simulink model "QPSK_HW_SW"  (R2017b)
settings: Solver=FixedStepDiscrete  StartTime=0.0  StopTime=inf  RelTol=1e-3
PreLoadFcn:
  | % Ensure SDR libraries are added to path
  | dev = sdrdev('PicoZed SDR');
  | dev.setupSession
  | clear dev; % clean up
  | 
  | sdrzQPSKTxFPGA_params = zynqRadioQPSKTxFPGAAD9361AD9364SL_init;
  | rcRolloff = 0.5;
  | sdrzQPSKrxFPGA = zynqRadioQPSKRxFPGAAD9361AD9364SL_init(rcRolloff);
  | % Need preamble & data from CST's QPSK Tx HDL example
  | qpsktxhdl=commqpsktxhdl_init();
  | 
  | % ARM Tx message
  | txtstr = '*Zynq HW/SW Codesign*';
InitFcn:
  | sdrzQPSKTxFPGA_params = zynqRadioQPSKTxFPGAAD9361AD9364SL_init;
  | rcRolloff = 0.5;
  | sdrzQPSKrxFPGA = zynqRadioQPSKRxFPGAAD9361AD9364SL_init(rcRolloff);
  | % Need preamble & data from CST's QPSK Tx HDL example
  | qpsktxhdl=commqpsktxhdl_init();
  | 
  | if (numel(txtstr) > 24)
  |   error('txtstr message must be less than 24 characters');
  | end;
undefined symbols (not defined in the file or in its folder): msglen
libraries: hdlsllib x15, dspsigops x6, commsequence2 x2, commdigbbndpm3 x2, dspmlti4 x2, commrandsrc3 x1, commutil2 x1, simulink x1, dspmathops x1
(part 1 of 2)
CloseFcn:
  | clear qpsktxhdl sdrzQPSKrxFPGA sdrzQPSKTxFPGA_params txtstr rcRolloff;
settings Model: DataTypeOverride=Off  Creator=The MathWorks, Inc.  LastModifiedBy=ppradhan
settings DataIOCC: SaveFormat=Array  SaveOutput=off  SaveTime=off
settings OptimizationCC: BlockReduction=off  ConditionallyExecuteInputs=off  DefaultParameterBehavior=Inlined  LifeSpan=inf
settings DebuggingCC: AlgebraicLoopMsg=error  SolverPrmCheckMsg=warning  SingleTaskRateTransMsg=error  ParameterPrecisionLossMsg=none  StrictBusMsg=ErrorOnBusTreatedAsVector  SFUnexpectedBacktrackingDiag=warning  SFNoUnconditionalDefaultTransitionDiag=warning  SFExecutionAtInitializationDiag=none
settings HardwareCC: ProdBitPerPointer=32  ProdBitPerSizeT=32  ProdBitPerPtrDiffT=32  ProdLargestAtomicFloat=None  ProdIntDivRoundTo=Undefined  ProdEndianess=Unspecified  ProdWordSize=32  ProdHWDeviceType=ASIC/FPGA->ASIC/FPGA  ProdEqTarget=off
settings ModelReferenceCC: PropagateSignalLabelsOutOfModel=off
settings CodeAppCC: StateflowObjectComments=on
settings GRTTargetCC: TargetLangStandard=C89/C90 (ANSI)  GeneratePreprocessorConditionals=Disable all
settings ConfigComp: CovMetricSettings=dw  CovHtmlReporting=on  CovSaveCumulativeToWorkspaceVar=on  CovSaveSingleToWorkspaceVar=on  CovExternalEMLEnable=off

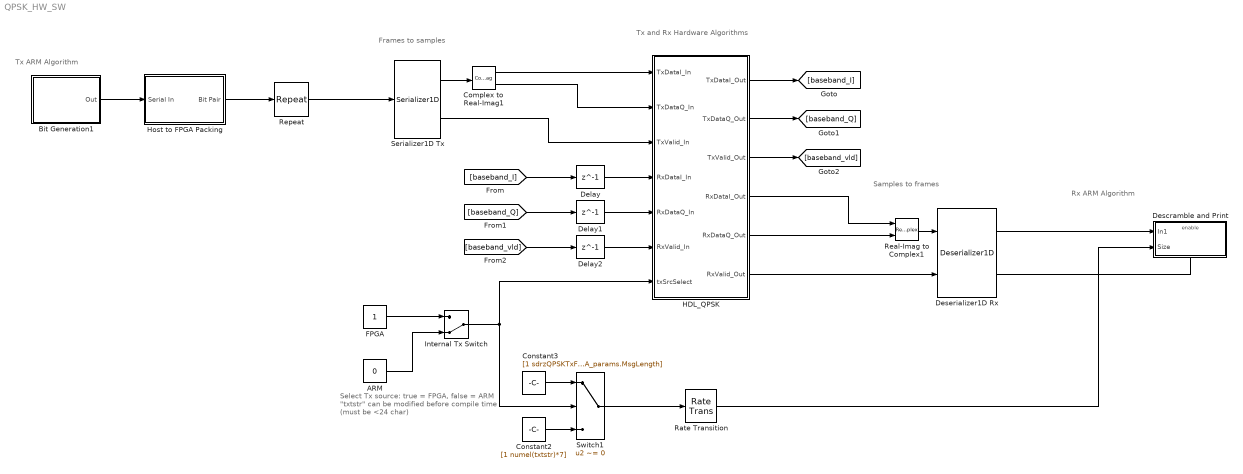
== system QPSK_HW_SW ==
  note: Select Tx source:
      | true = FPGA, false = ARM
      |
      | "txtstr" can be modified before
      | compile time (must be <24 char)
  note: Tx and Rx Hardware Algorithms
  note: Rx ARM Algorithm
  note: Samples to frames
  note: Frames to samples
  note: Tx ARM Algorithm
  ARM : Constant  Value=0  OutDataTypeStr=boolean  SampleTime=-1
  Bit Generation1 : Subsystem
      mask Display: disp('Bits Generation')
  Complex to Real-Imag1 : ComplexToRealImag
  Constant2 : Constant  Value=[1 numel(txtstr)*7]  SampleTime=-1
  Constant3 : Constant  Value=[1 sdrzQPSKTxFPGA_params.MsgLength]  SampleTime=-1
  Delay : Delay  DelayLength=1
  Delay1 : Delay  DelayLength=1
  Delay2 : Delay  DelayLength=1
  Descramble and Print : Subsystem  TreatAsAtomicUnit=on
  Deserializer1D Rx : hdlsllib/HDL Operations/Deserializer1D  Ratio=sdrzQPSKrxFPGA.FrameSize  IdleCycles=0  InitialCondition=0  startIn=off  validIn=on  validOut=on  inputDataDimensions=-1  inputSampleTime=-1  inputSignalType=auto
      settings: SourceProductName=HDL Coder  SourceProductBaseCode=HD
  FPGA : Constant  OutDataTypeStr=boolean  SampleTime=-1
  HDL_QPSK : Subsystem  TreatAsAtomicUnit=on
  Host to FPGA Packing : Subsystem
  Internal Tx Switch : ManualSwitch  CurrentSetting=0
  Rate Transition : RateTransition
  Real-Imag to Complex1 : RealImagToComplex
  Repeat : dspsigops/Repeat  N=4  InputProcessing=Columns as channels (frame based)  RateOptions=Allow multirate processing  ic=0  mode=Unused parameter value
      settings: SourceProductName=DSP System Toolbox
  Serializer1D Tx : hdlsllib/HDL Operations/Serializer1D  Ratio=200  IdleCycles=0  validIn=off  startOut=off  validOut=on  inputDataDimensions=-1  inputSampleTime=-1  inputSignalType=auto
      settings: SourceProductName=HDL Coder  SourceProductBaseCode=HD
  Switch1 : Switch  Criteria=u2 ~= 0
  wires:
  Deserializer1D Rx/1 -> Descramble and Print/1(In1)
  Real-Imag to Complex1/1 -> Deserializer1D Rx/1
  Deserializer1D Rx/2 -> Descramble and Print/Enable
  HDL_QPSK/4(RxDataI_Out) -> Real-Imag to Complex1/1
  HDL_QPSK/5(RxDataQ_Out) -> Real-Imag to Complex1/2
  HDL_QPSK/6(RxValid_Out) -> Deserializer1D Rx/2
  HDL_QPSK/1(TxDataI_Out) -> [baseband_I]
  HDL_QPSK/2(TxDataQ_Out) -> [baseband_Q]
  HDL_QPSK/3(TxValid_Out) -> [baseband_vld]
  [baseband_I] -> Delay/1
  [baseband_Q] -> Delay1/1
  [baseband_vld] -> Delay2/1
  Delay/1 -> HDL_QPSK/4(RxDataI_In)
  Delay1/1 -> HDL_QPSK/5(RxDataQ_In)
  Delay2/1 -> HDL_QPSK/6(RxValid_In)
  Host to FPGA Packing/1(Bit Pair) -> Repeat/1
  Bit Generation1/1(Out) -> Host to FPGA Packing/1(Serial In)
  Repeat/1 -> Serializer1D Tx/1
  Serializer1D Tx/1 -> Complex to Real-Imag1/1
  Complex to Real-Imag1/1 -> HDL_QPSK/1(TxDataI_In)
  Complex to Real-Imag1/2 -> HDL_QPSK/2(TxDataQ_In)
  Serializer1D Tx/2 -> HDL_QPSK/3(TxValid_In)
  ARM/1 -> Internal Tx Switch/2
  FPGA/1 -> Internal Tx Switch/1
  Switch1/1 -> Rate Transition/1
  Internal Tx Switch/1 -> HDL_QPSK/7(txSrcSelect), Switch1/2
  Constant2/1 -> Switch1/3
  Constant3/1 -> Switch1/1
  Rate Transition/1 -> Descramble and Print/2(Size)

== system QPSK_HW_SW/Bit Generation1 ==
  note: Each data frame contains 26 bits header (For Sync Purpose) and 174 bits data bits which
      | contain the txtStr message.Scrambler is there to improve data transition density and
      |  frequency offset estimation.
  Barker Code SS : Subsystem
      mask Display: disp('Unipolar\nBarker Code')
  Frame Conversion : FrameConversion  InheritSamplingMode=off  OutFrame=Sample-based
  Matrix Concatenate : Concatenate  Mode=Multidimensional array
  Message Source : Subsystem
      mask Display: disp('Message\nSource')
  Repeat : dspsigops/Repeat  N=2  InputProcessing=Columns as channels (frame based)  RateOptions=Enforce single-rate processing  ic=0  mode=Unused parameter value
      settings: SourceProductName=DSP System Toolbox
  Scrambler : commsequence2/Scrambler  M=2  poly=[1 1 1 0 1]  iniStaSource=Dialog Parameter  ini_sta=[0 0 0 0]  resetViaPort=off
      settings: SourceProductName=Communications System Toolbox  SourceProductBaseCode=CM
  Out : Outport
  wires:
  Message Source/1(Out) -> Scrambler/1
  Scrambler/1 -> Matrix Concatenate/2
  Repeat/1 -> Matrix Concatenate/1
  Barker Code SS/1(Out) -> Repeat/1
  Matrix Concatenate/1 -> Frame Conversion/1
  Frame Conversion/1 -> Out/1

== system QPSK_HW_SW/Descramble and Print ==
  In1 : Inport
  Size : Inport  Port=2
  Enable : EnablePort  PropagateVarSize=During execution
  BitsToDecimal1 : MATLAB Function  TreatAsAtomicUnit=on
  DataFramer : MATLAB Function  TreatAsAtomicUnit=on
  Descrambling : Subsystem
      mask Display: disp('Descrambling')
  wires:
  DataFramer/1(dataOut) -> Descrambling/1(In)
  In1/1 -> DataFramer/1(dataIn)
  Descrambling/1(Out) -> BitsToDecimal1/1(u)
  Size/1 -> Descrambling/2(Size)

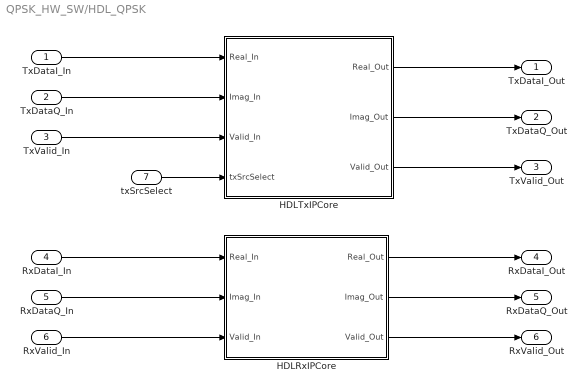
== system QPSK_HW_SW/HDL_QPSK ==
  TxDataI_In : Inport
  TxDataQ_In : Inport  Port=2
  TxValid_In : Inport  Port=3
  RxDataI_In : Inport  Port=4
  RxDataQ_In : Inport  Port=5
  RxValid_In : Inport  Port=6
  txSrcSelect : Inport  Port=7
  HDLRxIPCore : Subsystem  TreatAsAtomicUnit=on
  HDLTxIPCore : Subsystem  TreatAsAtomicUnit=on
  TxDataI_Out : Outport
  TxDataQ_Out : Outport  Port=2
  TxValid_Out : Outport  Port=3
  RxDataI_Out : Outport  Port=4
  RxDataQ_Out : Outport  Port=5
  RxValid_Out : Outport  Port=6
  wires:
  HDLTxIPCore/2(Imag_Out) -> TxDataQ_Out/1
  RxValid_In/1 -> HDLRxIPCore/3(Valid_In)
  HDLRxIPCore/3(Valid_Out) -> RxValid_Out/1
  HDLRxIPCore/2(Imag_Out) -> RxDataQ_Out/1
  HDLRxIPCore/1(Real_Out) -> RxDataI_Out/1
  HDLTxIPCore/3(Valid_Out) -> TxValid_Out/1
  RxDataQ_In/1 -> HDLRxIPCore/2(Imag_In)
  RxDataI_In/1 -> HDLRxIPCore/1(Real_In)
  HDLTxIPCore/1(Real_Out) -> TxDataI_Out/1
  TxDataI_In/1 -> HDLTxIPCore/1(Real_In)
  TxDataQ_In/1 -> HDLTxIPCore/2(Imag_In)
  TxValid_In/1 -> HDLTxIPCore/3(Valid_In)
  txSrcSelect/1 -> HDLTxIPCore/4(txSrcSelect)

== system QPSK_HW_SW/Host to FPGA Packing ==
  Serial In : Inport
  Data Type Conversion1 : DataTypeConversion  OutDataTypeStr=int16
  Downsample : DownSample  RateOptions=Allow multirate processing
  Downsample1 : DownSample  phase=1  RateOptions=Allow multirate processing
  Real-Imag to Complex : RealImagToComplex
  Bit Pair : Outport
  wires:
  Downsample/1 -> Real-Imag to Complex/1
  Serial In/1 -> Data Type Conversion1/1
  Data Type Conversion1/1 -> Downsample1/1, Downsample/1
  Downsample1/1 -> Real-Imag to Complex/2
  Real-Imag to Complex/1 -> Bit Pair/1

== system QPSK_HW_SW/Bit Generation1/Barker Code SS ==
  Constant Barker Code : Constant  Value=|  VectorParams1D=off  OutDataTypeStr=double
      | [+1 +1 +1 +1 +1 -1 -1 +1 +1 -1 +1 -1 +1
      | ].' > 0  % Bipolar to Unipolar Conversion
  Out : Outport
  wires:
  Constant Barker Code/1 -> Out/1

== system QPSK_HW_SW/Bit Generation1/Message Source ==
  Bernoulli Binary Generator : commrandsrc3/Bernoulli Binary Generator  ProbabilityOfZero=0.5  SeedSource=Parameter  Seed=61  SampleTime=sdrzQPSKTxFPGA_params.FrameTime / (sdrzQPSKTxFPGA_params.DataLength - numel(txtstr)*7)  SamplesPerFrame=sdrzQPSKTxFPGA_params.DataLength - numel(txtstr)*7  OutputDataType=double  SimulateUsing=Interpreted execution
  Integer to Bit Converter : commutil2/Integer to Bit Converter  nbits=7  signedInputValues=Unsigned  bitOrder=MSB first  outDtype=Inherit via internal rule
  Matrix Concatenate : Concatenate  Mode=Multidimensional array
  Scroll text : Constant  Value=double(txtstr)
  Out : Outport
  wires:
  Matrix Concatenate/1 -> Out/1
  Bernoulli Binary Generator/1 -> Matrix Concatenate/2
  Integer to Bit Converter/1 -> Matrix Concatenate/1
  Scroll text/1 -> Integer to Bit Converter/1

== system QPSK_HW_SW/Descramble and Print/Descrambling ==
  In : Inport
  Size : Inport  Port=2
  Descrambler : commsequence2/Descrambler  M=2  poly=[1 1 1 0 1]  iniStaSource=Dialog Parameter  ini_sta=[0 0 0 0]  resetViaPort=off
      settings: SourceProductName=Communications System Toolbox  SourceProductBaseCode=CM
  Selector : Selector  IndexOptions=Index vector (dialog)  Indices=[sdrzQPSKrxFPGA.BarkerLength*log2(sdrzQPSKrxFPGA.M)+1:sdrzQPSKrxFPGA.FrameSize*log2(sdrzQPSKrxFPGA.M)]  OutputSizes=1
  Selector1 : Selector  IndexOptions=Starting and ending indices (port)  Indices=[1:msglen]  OutputSizes=1
  Out : Outport
  wires:
  Selector/1 -> Descrambler/1
  In/1 -> Selector/1
  Selector1/1 -> Out/1
  Descrambler/1 -> Selector1/1
  Size/1 -> Selector1/2

== system QPSK_HW_SW/HDL_QPSK/HDLRxIPCore ==
  Real_In : Inport
  Imag_In : Inport  Port=2
  Valid_In : Inport  Port=3
  Complex to Real-Imag1 : ComplexToRealImag
  Enabled Delay : Delay  DelayLength=1  ShowEnablePort=on
      settings: InputPortMap=u0,e6
  HDLRx : Subsystem
  Real-Imag to Complex : RealImagToComplex
  Repeat : dspsigops/Repeat  N=sdrzQPSKrxFPGA.Upsampling/sdrzQPSKrxFPGA.Downsampling  InputProcessing=Columns as channels (frame based)  RateOptions=Allow multirate processing  ic=0  mode=Unused parameter value
      settings: SourceProductName=DSP System Toolbox
  Upsample : dspsigops/Upsample  N=sdrzQPSKrxFPGA.Upsampling/sdrzQPSKrxFPGA.Downsampling  phase=0  InputProcessing=Columns as channels (frame based)  RateOptions=Allow multirate processing  ic=0  mode=Unused parameter value
  Real_Out : Outport
  Imag_Out : Outport  Port=2
  Valid_Out : Outport  Port=3
  wires:
  HDLRx/2(dValidOut) -> Upsample/1
  Upsample/1 -> Valid_Out/1
  Repeat/1 -> Complex to Real-Imag1/1
  Complex to Real-Imag1/1 -> Real_Out/1
  Valid_In/1 -> Enabled Delay/2
  Complex to Real-Imag1/2 -> Imag_Out/1
  HDLRx/1(dataOutCh1) -> Repeat/1
  Real-Imag to Complex/1 -> Enabled Delay/1
  Enabled Delay/1 -> HDLRx/1(dataInCh1)
  Real_In/1 -> Real-Imag to Complex/1
  Imag_In/1 -> Real-Imag to Complex/2

== system QPSK_HW_SW/HDL_QPSK/HDLTxIPCore ==
  Real_In : Inport
  Imag_In : Inport  Port=2
  Valid_In : Inport  Port=3
  txSrcSelect : Inport  Port=4
  Complex to Real-Imag1 : ComplexToRealImag
  Delay : Delay  DelayLength=1
  Enabled Delay : Delay  DelayLength=1  ShowEnablePort=on
      settings: InputPortMap=u0,e6
  HDLTx : Subsystem
  Real-Imag to Complex : RealImagToComplex
  Real_Out : Outport
  Imag_Out : Outport  Port=2
  Valid_Out : Outport  Port=3
  wires:
  Complex to Real-Imag1/1 -> Real_Out/1
  Complex to Real-Imag1/2 -> Imag_Out/1
  HDLTx/1(dataoutCh1) -> Complex to Real-Imag1/1
  HDLTx/2(validoutCh1) -> Valid_Out/1
  Real-Imag to Complex/1 -> Enabled Delay/1
  Valid_In/1 -> HDLTx/2(validInCh1), Enabled Delay/2
  Real_In/1 -> Real-Imag to Complex/1
  Imag_In/1 -> Real-Imag to Complex/2
  Enabled Delay/1 -> HDLTx/1(dataInCh1)
  txSrcSelect/1 -> Delay/1
  Delay/1 -> HDLTx/3(txSrcSelect)

== system QPSK_HW_SW/HDL_QPSK/HDLRxIPCore/HDLRx ==
  dataInCh1 : Inport
  Automatic Gain Control : Subsystem  mask{AGCLoopGain=0.1, AGCUpperLimit=400, AGCRef=1/sqrt(sdrzQPSKrxFPGA.Upsampling)}
      mask prompts: AGCLoopGain "Loop Gain"; AGCUpperLimit "Maximum Gain"; AGCRef "Desired Amplitude"
  Coarse Frequency Compensation : Subsystem
  Data Decoding : Subsystem  TreatAsAtomicUnit=on  mask{Threshold=16}
      mask help:
      | Package synchronization is achieved by correlating (matched filtering) the Barker codes with the streams given by the Timing Recovery subsystem.
      | We deem successful package synchronization if the modulus of the matched filter output exceeds the threshold value defined below.
  FPGA to Host : Subsystem
  Fine Frequency Compensation : Subsystem
  Logical Operator1 : Logic  AllPortsSameDT=off  OutDataTypeStr=boolean
  Root Raised Cosine Receive Filter : dspmlti4/FIR Decimation  FilterSource=Dialog parameters  h=sdrzQPSKrxFPGA.rcRxFilt  D=sdrzQPSKrxFPGA.Upsampling/sdrzQPSKrxFPGA.Downsampling  filtStruct=Direct form  FilterObject=Hm_firdecim  framing=Allow multirate processing  inputOffset=0  outputBufInitCond=0  roundingMode=Floor  overflowMode=off  firstCoeffDataTypeStr=Inherit: Same word length as input  firstCoeffMin=[]  firstCoeffMax=[]  firstCoeffLastDataTypeStr=Inherit: Same word length as input  prodOutputMode=Binary point scaling  prodOutputWordLength=31  prodOutputFracLength=29  prodOutputDataTypeStr=fixdt(1,31,29)  prodOutputLastDataTypeStr=fixdt(1,31,29)  accumMode=Binary point scaling  accumWordLength=33  accumFracLength=29  accumDataTypeStr=fixdt(1,33,29)  accumLastDataTypeStr=fixdt(1,33,29)  outputMode=Binary point scaling  outputWordLength=16  outputFracLength=14  outputDataTypeStr=fixdt(1,16,14)  outputMin=[]  outputMax=[]  outputLastDataTypeStr=fixdt(1,16,14)
  Timing Recovery : Subsystem
  dataOutCh1 : Outport
  dValidOut : Outport  Port=2
  wires:
  FPGA to Host/1(Out) -> dataOutCh1/1
  Timing Recovery/2(DataOut) -> Data Decoding/1(In)
  dataInCh1/1 -> Automatic Gain Control/1(In)
  Fine Frequency Compensation/1(Out) -> Timing Recovery/1(In)
  Coarse Frequency Compensation/1(Out) -> Fine Frequency Compensation/1(In)
  Timing Recovery/1(dValid) -> Data Decoding/Enable, Logical Operator1/1
  Data Decoding/2(Bit1) -> FPGA to Host/1(bit1)
  Data Decoding/1(dValid) -> Logical Operator1/2
  Root Raised Cosine Receive Filter/1 -> Coarse Frequency Compensation/1(In)
  Automatic Gain Control/1(Out) -> Root Raised Cosine Receive Filter/1
  Logical Operator1/1 -> dValidOut/1
  Data Decoding/3(Bit2) -> FPGA to Host/2(bit2)

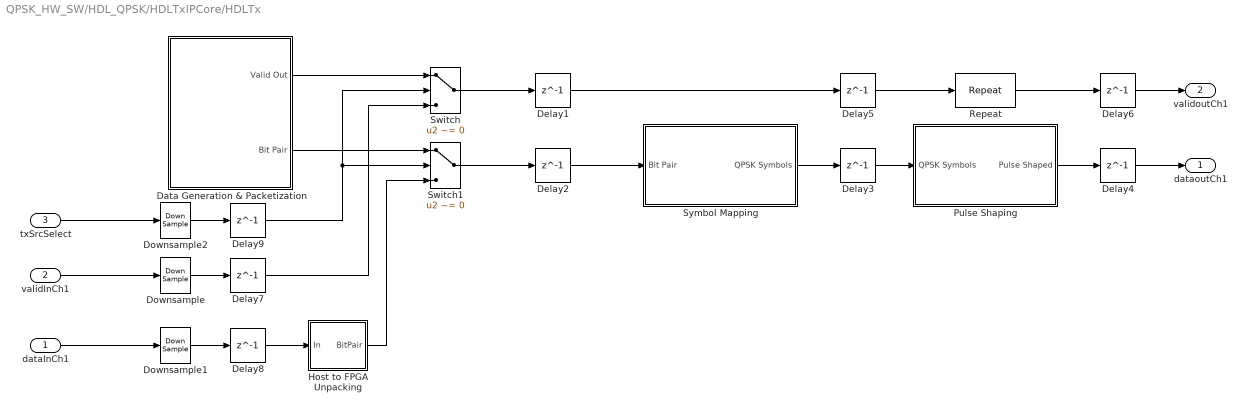
== system QPSK_HW_SW/HDL_QPSK/HDLTxIPCore/HDLTx ==
  dataInCh1 : Inport
  validInCh1 : Inport  Port=2
  txSrcSelect : Inport  Port=3
  Data Generation & Packetization : Subsystem
  Delay{1..9} (9 alike) : Delay  DelayLength=1  InitialCondition=0
  Downsample : DownSample  N=sdrzQPSKTxFPGA_params.Upsampling  RateOptions=Allow multirate processing
  Downsample1 : DownSample  N=sdrzQPSKTxFPGA_params.Upsampling  RateOptions=Allow multirate processing
  Downsample2 : DownSample  N=sdrzQPSKTxFPGA_params.Upsampling  RateOptions=Allow multirate processing
  Host to FPGA Unpacking : Subsystem
  Pulse Shaping : Subsystem
  Repeat : dspsigops/Repeat  N=sdrzQPSKTxFPGA_params.Upsampling  InputProcessing=Columns as channels (frame based)  RateOptions=Allow multirate processing  ic=0  mode=Unused parameter value
      settings: SourceProductName=DSP System Toolbox
  Switch : Switch  Criteria=u2 ~= 0
  Switch1 : Switch  Criteria=u2 ~= 0
  Symbol Mapping : Subsystem
  dataoutCh1 : Outport
  validoutCh1 : Outport  Port=2
  wires:
  Delay3/1 -> Pulse Shaping/1(QPSK Symbols)
  Pulse Shaping/1(Pulse Shaped) -> Delay4/1
  Delay4/1 -> dataoutCh1/1
  Delay2/1 -> Symbol Mapping/1(Bit Pair)
  Symbol Mapping/1(QPSK Symbols) -> Delay3/1
  Delay1/1 -> Delay5/1
  Delay5/1 -> Repeat/1
  Repeat/1 -> Delay6/1
  Delay6/1 -> validoutCh1/1
  Data Generation & Packetization/1(Valid Out) -> Switch/1
  Data Generation & Packetization/2(Bit Pair) -> Switch1/1
  Switch/1 -> Delay1/1
  Switch1/1 -> Delay2/1
  Downsample/1 -> Delay7/1
  Downsample1/1 -> Delay8/1
  validInCh1/1 -> Downsample/1
  dataInCh1/1 -> Downsample1/1
  Delay8/1 -> Host to FPGA Unpacking/1(In)
  Host to FPGA Unpacking/1(BitPair) -> Switch1/3
  Delay7/1 -> Switch/3
  Downsample2/1 -> Delay9/1
  txSrcSelect/1 -> Downsample2/1
  Delay9/1 -> Switch/2, Switch1/2

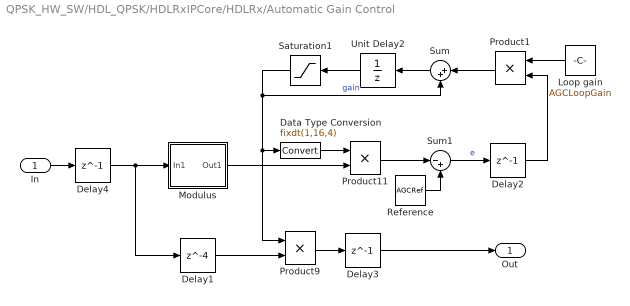
== system QPSK_HW_SW/HDL_QPSK/HDLRxIPCore/HDLRx/Automatic Gain Control ==
  In : Inport
  Data Type Conversion : DataTypeConversion  OutDataTypeStr=fixdt(1,16,4)  SaturateOnIntegerOverflow=on
  Delay1 : Delay  DelayLength=4  InitialCondition=0
  Delay2 : Delay  DelayLength=1  InitialCondition=0
  Delay3 : Delay  DelayLength=1  InitialCondition=0
  Delay4 : Delay  DelayLength=1  InitialCondition=0
  Loop gain : Constant  Value=AGCLoopGain  OutDataTypeStr=fixdt(1,16,10)  SampleTime=sdrzQPSKrxFPGA.Ts
  Modulus : Subsystem
  Product1 : Product  OutDataTypeStr=fixdt(1,16,10)  RndMeth=Zero
  Product11 : Product  OutDataTypeStr=fixdt(1,16,10)  RndMeth=Zero
  Product9 : Product  OutDataTypeStr=fixdt(1,16,14)  SaturateOnIntegerOverflow=on  RndMeth=Zero
  Reference : Constant  Value=AGCRef  OutDataTypeStr=fixdt(1,16,10)  SampleTime=sdrzQPSKrxFPGA.Ts
  Saturation1 : Saturate  UpperLimit=AGCUpperLimit  LowerLimit=1e-5
  Sum : Sum  Inputs=|++  OutDataTypeStr=fixdt(1,23,10)  SaturateOnIntegerOverflow=on
  Sum1 : Sum  Inputs=|-+  OutDataTypeStr=Inherit: Same as first input
  Unit Delay2 : UnitDelay  SampleTime=-1
  Out : Outport  PortDimensions=1
  wires:
  In/1 -> Delay4/1
  Product11/1 -> Sum1/1
  Data Type Conversion/1 -> Product11/1
  Reference/1 -> Sum1/2
  Sum/1 -> Unit Delay2/1
  Sum1/1 -> Delay2/1  "e"
  Product9/1 -> Delay3/1
  Delay1/1 -> Product9/2
  Delay3/1 -> Out/1
  Delay2/1 -> Product1/2
  Unit Delay2/1 -> Saturation1/1
  Delay4/1 -> Delay1/1, Modulus/1(In1)
  Modulus/1(Out1) -> Product11/2
  Product1/1 -> Sum/1
  Loop gain/1 -> Product1/1
  Saturation1/1 -> Data Type Conversion/1, Product9/1, Sum/2  "gain"

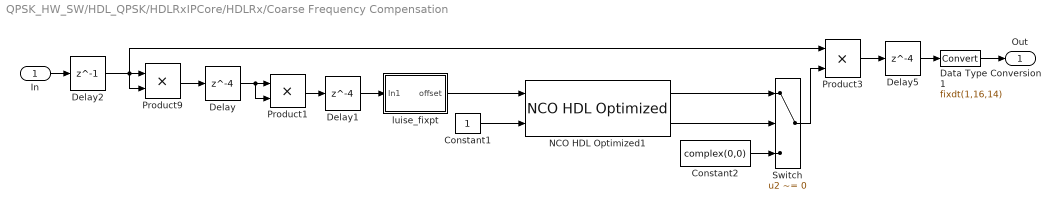
== system QPSK_HW_SW/HDL_QPSK/HDLRxIPCore/HDLRx/Coarse Frequency Compensation ==
  In : Inport  PortDimensions=1
  Constant1 : Constant  OutDataTypeStr=boolean  SampleTime=sdrzQPSKrxFPGA.Ts*sdrzQPSKrxFPGA.Upsampling/sdrzQPSKrxFPGA.Downsampling
  Constant2 : Constant  Value=complex(0,0)  OutDataTypeStr=fixdt(1,10,8)  SampleTime=sdrzQPSKrxFPGA.Ts*sdrzQPSKrxFPGA.Upsampling/sdrzQPSKrxFPGA.Downsampling
  Data Type Conversion1 : DataTypeConversion  OutDataTypeStr=fixdt(1,16,14)
  Delay : Delay  DelayLength=4  InitialCondition=0
  Delay1 : Delay  DelayLength=4  InitialCondition=0
  Delay2 : Delay  DelayLength=1  InitialCondition=0
  Delay5 : Delay  DelayLength=4  InitialCondition=0
  NCO HDL Optimized1 : dspsigops/NCO HDL Optimized  PhaseIncrementSource=Input port  PhaseIncrement=100  PhaseOffsetSource=Property  PhaseOffset=0  DitherSource=None  NumDitherBits=1  PhaseQuantization=on  NumQuantizerAccumulatorBits=16  LUTCompress=on  ResetAction=off  ValidInputPort=on  Waveform=Complex exponential  PhasePort=off  SimulateUsing=Code generation  AccumulatorWL=17  OutputDataType=Binary point scaling  OutputWL=10  OutputFL=8
      settings: SourceProductName=DSP System Toolbox  SourceProductBaseCode=DS
  Product1 : Product  SaturateOnIntegerOverflow=on  RndMeth=Zero
  Product3 : Product  SaturateOnIntegerOverflow=on  RndMeth=Zero
  Product9 : Product  OutDataTypeStr=fixdt(1,16,13)  SaturateOnIntegerOverflow=on  RndMeth=Zero
  Switch : Switch  Criteria=u2 ~= 0
  luise_fixpt : Subsystem
  Out : Outport
  wires:
  Data Type Conversion1/1 -> Out/1
  luise_fixpt/1(offset) -> NCO HDL Optimized1/1
  Delay1/1 -> luise_fixpt/1(In1)
  Product9/1 -> Delay/1
  Delay/1 -> Product1/1, Product1/2
  Product1/1 -> Delay1/1
  In/1 -> Delay2/1
  Product3/1 -> Delay5/1
  Delay5/1 -> Data Type Conversion1/1
  Constant1/1 -> NCO HDL Optimized1/2
  NCO HDL Optimized1/2 -> Switch/2
  NCO HDL Optimized1/1 -> Switch/1
  Constant2/1 -> Switch/3
  Switch/1 -> Product3/2
  Delay2/1 -> Product3/1, Product9/2, Product9/1

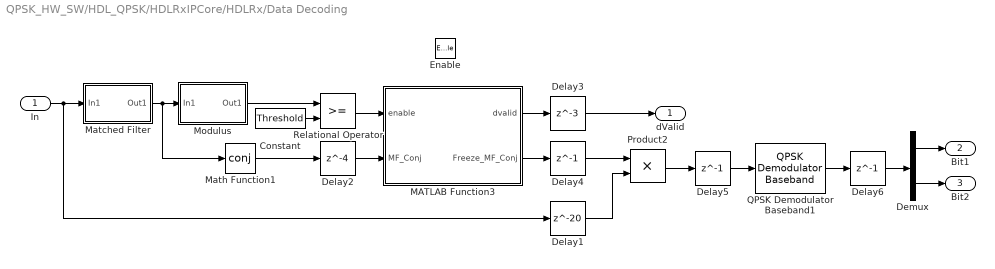
== system QPSK_HW_SW/HDL_QPSK/HDLRxIPCore/HDLRx/Data Decoding ==
  In : Inport
  Enable : EnablePort
  Constant : Constant  Value=Threshold  OutDataTypeStr=Inherit: Inherit via back propagation  SampleTime=sdrzQPSKrxFPGA.Ts*sdrzQPSKrxFPGA.Upsampling/sdrzQPSKrxFPGA.Downsampling
  Delay1 : Delay  DelayLength=20  InitialCondition=0
  Delay2 : Delay  DelayLength=4  InitialCondition=0
  Delay3 : Delay  DelayLength=3  InitialCondition=0
  Delay4 : Delay  DelayLength=1  InitialCondition=0
  Delay5 : Delay  DelayLength=1  InitialCondition=0
  Delay6 : Delay  DelayLength=1  InitialCondition=0
  Demux : Demux  Outputs=2
  MATLAB Function3 : MATLAB Function  TreatAsAtomicUnit=on
  Matched Filter : Subsystem
  Math Function1 : Math  Operator=conj  OutputSignalType=complex  SaturateOnIntegerOverflow=on
  Modulus : Subsystem
  Product2 : Product  SaturateOnIntegerOverflow=on  RndMeth=Zero
  QPSK Demodulator Baseband1 : commdigbbndpm3/QPSK Demodulator Baseband  OutType=Bit  DecType=Hard decision  VarSource=Dialog  Variance=1  Dec=Gray  Ph=pi/4  outDtype1=boolean  outDtype2=Inherit via internal rule  derotateFactorWordLen=16  derotateFactorDataTypeStr=Inherit: Same word length as input  derotateFactorLastDataTypeStr=Inherit: Same word length as input
  Relational Operator : RelationalOperator  OutDataTypeStr=boolean  RndMeth=Nearest  InputSameDT=on
  dValid : Outport  InitialOutput=0
  Bit1 : Outport  Port=2  InitialOutput=0
  Bit2 : Outport  Port=3  InitialOutput=0
  wires:
  Demux/2 -> Bit2/1
  Demux/1 -> Bit1/1
  Delay3/1 -> dValid/1
  Delay6/1 -> Demux/1
  Delay5/1 -> QPSK Demodulator Baseband1/1
  Delay1/1 -> Product2/2
  Delay4/1 -> Product2/1
  Delay2/1 -> MATLAB Function3/2(MF_Conj)
  Matched Filter/1(Out1) -> Math Function1/1, Modulus/1(In1)
  In/1 -> Delay1/1, Matched Filter/1(In1)
  Relational Operator/1 -> MATLAB Function3/1(enable)
  Math Function1/1 -> Delay2/1
  MATLAB Function3/2(Freeze_MF_Conj) -> Delay4/1
  MATLAB Function3/1(dvalid) -> Delay3/1
  QPSK Demodulator Baseband1/1 -> Delay6/1
  Modulus/1(Out1) -> Relational Operator/1
  Constant/1 -> Relational Operator/2
  Product2/1 -> Delay5/1

== system QPSK_HW_SW/HDL_QPSK/HDLRxIPCore/HDLRx/FPGA to Host ==
  bit1 : Inport
  bit2 : Inport  Port=2
  Data Type Conversion1 : DataTypeConversion  OutDataTypeStr=int16
  Data Type Conversion2 : DataTypeConversion  OutDataTypeStr=int16
  Real-Imag to Complex : RealImagToComplex
  Out : Outport
  wires:
  Data Type Conversion1/1 -> Real-Imag to Complex/1
  Real-Imag to Complex/1 -> Out/1
  bit2/1 -> Data Type Conversion2/1
  Data Type Conversion2/1 -> Real-Imag to Complex/2
  bit1/1 -> Data Type Conversion1/1

== system QPSK_HW_SW/HDL_QPSK/HDLRxIPCore/HDLRx/Fine Frequency Compensation ==
  In : Inport  PortDimensions=1
  Delay2 : Delay  InitialCondition=0
  Loop Filter : Subsystem  mask{BnTs=0.13, zeta=2.5, N=sdrzQPSKrxFPGA.Upsampling/sdrzQPSKrxFPGA.Downsampling}
      mask prompts: BnTs "Normalized Loop Bandwidth"; zeta "Damping Factor"; N "Number of Samples/Symbol"
      mask init:
      | % See C.57 to C.61 in Michael Rice's "Digital Communications 
      | % - A Discrete-Time Approach" for details
      | 
      | theta = BnTs/(zeta+0.25/zeta);  %0.0385
      | d = 1 + 2*zeta*theta + theta*theta; %1.1938
      | K1 = zeta*theta/d; %0.0805
      | K2 = theta*theta/(d*2); %6.1958e-04
      mask Display: disp('Loop Filter')
  MATLAB Function1 : MATLAB Function  TreatAsAtomicUnit=on
  Phase Calculation : Subsystem
  Product : Product  SaturateOnIntegerOverflow=on  OutDataTypeStr=Inherit: Same as first input
  Out : Outport
  wires:
  In/1 -> Product/1
  Loop Filter/1(v) -> Phase Calculation/1(Inc)
  MATLAB Function1/1(e) -> Loop Filter/1(e)
  Product/1 -> Delay2/1
  Delay2/1 -> MATLAB Function1/1(In), Out/1
  Phase Calculation/1(phShift) -> Product/2

== system QPSK_HW_SW/HDL_QPSK/HDLRxIPCore/HDLRx/Timing Recovery ==
  In : Inport
  Delay5 : Delay  DelayLength=6
  Integer Delay3 : Delay  DelayLength=1  InputProcessing=Inherited
  Integer Delay4 : Delay  DelayLength=1  InputProcessing=Inherited
  Interpolation Control : MATLAB Function
  Interpolation Filter : Subsystem
  Loop Filter : Subsystem  mask{BnTs=0.01, zeta=1, Kp=sdrzQPSKrxFPGA.TimingRecTEDGain, K0=sdrzQPSKrxFPGA.TimingRecCompensateGain, N=sdrzQPSKrxFPGA.Upsampling/sdrzQPSKrxFPGA.Downsampling}
      mask prompts: BnTs "Loop Bandwidth"; zeta "Loop Damping Factor"; Kp "Phase Detector Gain (Kp)"; K0 "DDS gain (K0)"; N "Number of Samples/symbol (N)"
      mask init:
      | % See C.57 to C.61 in Michael Rice's "Digital Communications 
      | % - A Discrete-Time Approach" for details
      | theta = BnTs/(zeta+0.25/zeta)/N;
      | d = 1 + 2*zeta*theta + theta*theta;
      | K1 = 4*zeta*theta/d;
      | K2 = 4*theta*theta/d;
      | K1 = K1/(Kp*K0);
      | K2 = K2/(Kp*K0);
      mask Display: disp('Loop Filter');
  Timing Error Detector : MATLAB Function  TreatAsAtomicUnit=on
  dValid : Outport
  DataOut : Outport  Port=2
  wires:
  Interpolation Filter/1(Out) -> Timing Error Detector/1(In), DataOut/1
  In/1 -> Delay5/1
  Integer Delay4/1 -> Interpolation Filter/2(mu)
  Interpolation Control/2(mu) -> Integer Delay4/1
  Interpolation Control/1(Underflow) -> Integer Delay3/1
  Delay5/1 -> Interpolation Filter/1(In)
  Integer Delay3/1 -> dValid/1, Timing Error Detector/2(strobe)
  Timing Error Detector/1(e) -> Loop Filter/1(e)
  Loop Filter/1(v) -> Interpolation Control/1(Delta)

== system QPSK_HW_SW/HDL_QPSK/HDLTxIPCore/HDLTx/Data Generation & Packetization ==
  Bit Pairing : Subsystem
  Data Source : Subsystem
  Downsample : DownSample  RateOptions=Allow multirate processing
  PacketizerFSM : MATLAB Function  TreatAsAtomicUnit=on  SystemSampleTime=1/sdrzQPSKrxFPGA.RadioFrontEndSampleRate*2
  Pipeline : Delay  InitialCondition=0
  Pipeline1 : Delay  DelayLength=1  InitialCondition=0
  Pipeline2 : Delay  DelayLength=1  InitialCondition=0
  Pipeline3 : Delay  DelayLength=1  InitialCondition=0
  Valid : Constant  OutDataTypeStr=boolean  SampleTime=1/sdrzQPSKrxFPGA.RadioFrontEndSampleRate*2
  Valid Out : Outport
  Bit Pair : Outport  Port=2
  wires:
  Bit Pairing/1(Bit Pair) -> Bit Pair/1
  Pipeline2/1 -> Bit Pairing/1(Serial In)
  Data Source/1(packets) -> Pipeline2/1
  Valid/1 -> Pipeline/1
  Pipeline1/1 -> Downsample/1
  Pipeline/1 -> Pipeline1/1
  Downsample/1 -> Pipeline3/1
  Pipeline3/1 -> Valid Out/1
  PacketizerFSM/1(reset_preamble) -> Data Source/1(reset preamble)
  PacketizerFSM/2(load_preamble) -> Data Source/2(load preamble)
  PacketizerFSM/3(load_data) -> Data Source/3(load data)

== system QPSK_HW_SW/HDL_QPSK/HDLTxIPCore/HDLTx/Host to FPGA Unpacking ==
  In : Inport
  Bit Concat : hdlsllib/HDL Operations/Bit Concat  numInputs=2
      settings: SourceProductName=HDL Coder  SourceProductBaseCode=HD
  Bit Slice1 : hdlsllib/HDL Operations/Bit Slice  lidx=0  ridx=0
      settings: SourceProductName=HDL Coder  SourceProductBaseCode=HD
  Bit Slice2 : hdlsllib/HDL Operations/Bit Slice  lidx=0  ridx=0
      settings: SourceProductName=HDL Coder  SourceProductBaseCode=HD
  Complex to Real-Imag : ComplexToRealImag
  BitPair : Outport
  wires:
  Complex to Real-Imag/1 -> Bit Slice2/1
  Complex to Real-Imag/2 -> Bit Slice1/1
  Bit Slice2/1 -> Bit Concat/1
  Bit Slice1/1 -> Bit Concat/2
  Bit Concat/1 -> BitPair/1
  In/1 -> Complex to Real-Imag/1

== system QPSK_HW_SW/HDL_QPSK/HDLTxIPCore/HDLTx/Pulse Shaping ==
  QPSK Symbols : Inport
  RRC Interpolation Filter : dspmlti4/FIR Interpolation  FilterSource=Dialog parameters  h=sdrzQPSKTxFPGA_params.TransmitterFilterCoefficients  L=sdrzQPSKTxFPGA_params.Upsampling  FilterObject=Htxrc  framing=Allow multirate processing  outputBufInitCond=0  roundingMode=Floor  overflowMode=off  firstCoeffMode=Specify word length  firstCoeffWordLength=16  firstCoeffFracLength=15  firstCoeffDataTypeStr=fixdt(1,16)  firstCoeffMin=[]  firstCoeffMax=[]  firstCoeffLastDataTypeStr=fixdt(1,16)  prodOutputMode=Binary point scaling  prodOutputWordLength=31  prodOutputFracLength=29  prodOutputDataTypeStr=fixdt(1,31,29)  prodOutputLastDataTypeStr=fixdt(1,31,29)  accumMode=Binary point scaling  accumWordLength=33  accumFracLength=29  accumDataTypeStr=fixdt(1,33,29)  accumLastDataTypeStr=fixdt(1,33,29)  outputMode=Binary point scaling  outputWordLength=16  outputFracLength=14  outputDataTypeStr=fixdt(1,16,14)  outputMin=[]  outputMax=[]  outputLastDataTypeStr=fixdt(1,16,14)
      settings: SourceProductName=DSP System Toolbox
  Pulse Shaped : Outport
  wires:
  QPSK Symbols/1 -> RRC Interpolation Filter/1
  RRC Interpolation Filter/1 -> Pulse Shaped/1

== system QPSK_HW_SW/HDL_QPSK/HDLTxIPCore/HDLTx/Symbol Mapping ==
  Bit Pair : Inport
  QPSK Modulator Baseband : commdigbbndpm3/QPSK Modulator Baseband  InType=Integer  Enc=Gray  Ph=pi/4  outDtype=Fixed-point  outWordLen=16  outUDDataType=sfix(16)  outFracLenMode=User-defined  outFracLen=15  outDataTypeStr=fixdt(1,16,15)  outLastDataTypeStr=fixdt(1,16,15)
  QPSK Symbols : Outport
  wires:
  QPSK Modulator Baseband/1 -> QPSK Symbols/1
  Bit Pair/1 -> QPSK Modulator Baseband/1

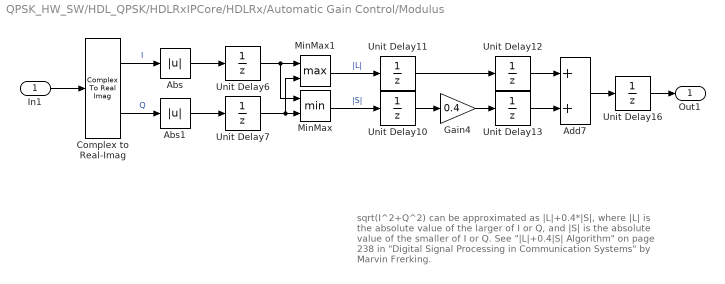
== system QPSK_HW_SW/HDL_QPSK/HDLRxIPCore/HDLRx/Automatic Gain Control/Modulus ==
  note: sqrt(I^2+Q^2) can be approximated as |L|+0.4*|S|,
      | where |L| is the absolute value of the larger of I or Q,
      | and |S| is the absolute value of the smaller of I or Q.
      |
      | See "|L|+0.4|S| Algorithm" on page 238 in "Digital Signal
      | Processing in Communication Systems" by Marvin Frerking.
  In1 : Inport
  Abs : Abs
  Abs1 : Abs
  Add7 : Sum
  Complex to Real-Imag : ComplexToRealImag
  Gain4 : Gain  Gain=0.4  OutDataTypeStr=fixdt(1,16,15)
  MinMax : MinMax  Inputs=2
  MinMax1 : MinMax  Function=max  Inputs=2
  Unit Delay{6..7,10..13,16} (7 alike) : UnitDelay  SampleTime=-1
  Out1 : Outport
  wires:
  Unit Delay11/1 -> Unit Delay12/1
  Unit Delay16/1 -> Out1/1
  Unit Delay10/1 -> Gain4/1
  Unit Delay12/1 -> Add7/1
  Abs1/1 -> Unit Delay7/1
  Add7/1 -> Unit Delay16/1
  Abs/1 -> Unit Delay6/1
  Complex to Real-Imag/1 -> Abs/1  "I"
  Complex to Real-Imag/2 -> Abs1/1  "Q"
  MinMax1/1 -> Unit Delay11/1  "|L|"
  Unit Delay13/1 -> Add7/2
  Gain4/1 -> Unit Delay13/1
  MinMax/1 -> Unit Delay10/1  "|S|"
  Unit Delay6/1 -> MinMax/1, MinMax1/1
  Unit Delay7/1 -> MinMax1/2, MinMax/2
  In1/1 -> Complex to Real-Imag/1

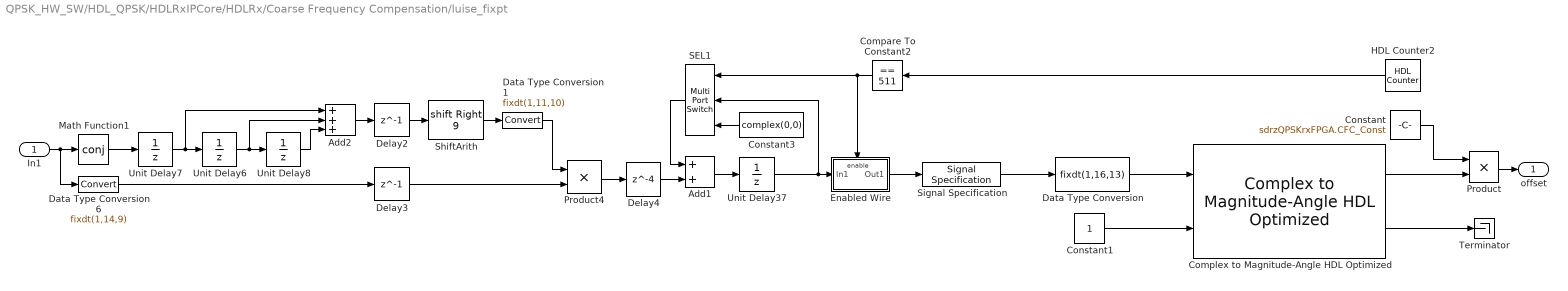
== system QPSK_HW_SW/HDL_QPSK/HDLRxIPCore/HDLRx/Coarse Frequency Compensation/luise_fixpt ==
  In1 : Inport
  Add1 : Sum  OutDataTypeStr=fixdt(1,33,20)
  Add2 : Sum  Inputs=+++  OutDataTypeStr=fixdt(1,33,20)
  Compare To Constant2 : simulink/Logic and Bit Operations/Compare To Constant  relop===  const=511  OutDataTypeStr=boolean
  Complex to Magnitude-Angle HDL Optimized : dspmathops/Complex to Magnitude-Angle HDL Optimized  NumIterationsSource=Property  NumIterations=5  OutputFormat=Angle  AngleFormat=Normalized  ScaleOutput=on  SimulateUsing=Code generation
      settings: SourceProductName=DSP System Toolbox  SourceProductBaseCode=DS
  Constant : Constant  Value=sdrzQPSKrxFPGA.CFC_Const  OutDataTypeStr=int16  SampleTime=sdrzQPSKrxFPGA.Ts*sdrzQPSKrxFPGA.Upsampling/sdrzQPSKrxFPGA.Downsampling
  Constant1 : Constant  OutDataTypeStr=boolean  SampleTime=sdrzQPSKrxFPGA.Ts*sdrzQPSKrxFPGA.Upsampling/sdrzQPSKrxFPGA.Downsampling
  Constant3 : Constant  Value=complex(0,0)  OutDataTypeStr=fixdt(1,16,14)  SampleTime=sdrzQPSKrxFPGA.Ts*sdrzQPSKrxFPGA.Upsampling/sdrzQPSKrxFPGA.Downsampling
  Data Type Conversion : DataTypeConversion  OutDataTypeStr=fixdt(1,16,13)
  Data Type Conversion1 : DataTypeConversion  OutDataTypeStr=fixdt(1,11,10)
  Data Type Conversion6 : DataTypeConversion  OutDataTypeStr=fixdt(1,14,9)  SaturateOnIntegerOverflow=on
  Delay2 : Delay  DelayLength=1  InitialCondition=0
  Delay3 : Delay  DelayLength=1  InitialCondition=0
  Delay4 : Delay  DelayLength=4  InitialCondition=0
  Enabled Wire : Subsystem  TreatAsAtomicUnit=on
  HDL Counter2 : hdlsllib/HDL Operations/HDL Counter  CountType=Count limited  CountInit=0  CountStep=1  CountMax=511  CountFromType=Initial value  CountFrom=0  CountResetPort=off  CountLoadPort=off  CountEnbPort=off  CountDirPort=off  CountDataType=Unsigned  CountWordLen=9  CountFracLen=0  CountSampTime=sdrzQPSKrxFPGA.Ts*sdrzQPSKrxFPGA.Upsampling/sdrzQPSKrxFPGA.Downsampling
      settings: SourceProductName=HDL Coder  SourceProductBaseCode=HD
  Math Function1 : Math  Operator=conj  OutputSignalType=complex  SaturateOnIntegerOverflow=on
  Product : Product  OutDataTypeStr=int16
  Product4 : Product  SaturateOnIntegerOverflow=on  RndMeth=Zero
  SEL1 : MultiPortSwitch  DataPortOrder=Zero-based contiguous  Inputs=2  DiagnosticForDefault=None  OutDataTypeStr=fixdt(1,33,20)
  ShiftArith : ArithShift  BitShiftNumber=9  BitShiftDirection=Right
  Signal Specification : SignalSpecification  Dimensions=1
  Terminator : Terminator
  Unit Delay37 : UnitDelay  InitialCondition=0+0j  SampleTime=-1
  Unit Delay6 : UnitDelay  SampleTime=-1
  Unit Delay7 : UnitDelay  SampleTime=-1
  Unit Delay8 : UnitDelay  SampleTime=-1
  offset : Outport  PortDimensions=1
  wires:
  Delay2/1 -> ShiftArith/1
  Delay3/1 -> Product4/2
  ShiftArith/1 -> Data Type Conversion1/1
  Unit Delay8/1 -> Add2/3
  HDL Counter2/1 -> Compare To Constant2/1
  Compare To Constant2/1 -> SEL1/1, Enabled Wire/Enable
  Unit Delay7/1 -> Unit Delay6/1, Add2/1
  Unit Delay6/1 -> Add2/2, Unit Delay8/1
  Constant3/1 -> SEL1/3
  Data Type Conversion6/1 -> Delay3/1
  Add2/1 -> Delay2/1
  SEL1/1 -> Add1/1
  Unit Delay37/1 -> SEL1/2, Enabled Wire/1(In1)
  Delay4/1 -> Add1/2
  Data Type Conversion1/1 -> Product4/1
  In1/1 -> Data Type Conversion6/1, Math Function1/1
  Product4/1 -> Delay4/1
  Math Function1/1 -> Unit Delay7/1
  Add1/1 -> Unit Delay37/1
  Enabled Wire/1(Out1) -> Signal Specification/1
  Product/1 -> offset/1
  Constant/1 -> Product/1
  Complex to Magnitude-Angle HDL Optimized/1 -> Product/2
  Constant1/1 -> Complex to Magnitude-Angle HDL Optimized/2
  Signal Specification/1 -> Data Type Conversion/1
  Complex to Magnitude-Angle HDL Optimized/2 -> Terminator/1
  Data Type Conversion/1 -> Complex to Magnitude-Angle HDL Optimized/1

== system QPSK_HW_SW/HDL_QPSK/HDLRxIPCore/HDLRx/Data Decoding/Matched Filter ==
  In1 : Inport
  Add2 : Sum
  Add3 : Sum  Inputs=+-
  Complex to Real-Imag2 : ComplexToRealImag
  Data Type Conversion1 : DataTypeConversion  OutDataTypeStr=fixdt(1,16,10)
  Data Type Conversion6 : DataTypeConversion  OutDataTypeStr=fixdt(1,16,10)
  Delay{1..4} (4 alike) : Delay  DelayLength=1  InitialCondition=0
  Discrete FIR Filter3 : DiscreteFir  FilterStructure=Direct form transposed  Coefficients=[-1 1 -1 1 -1 -1 1 1 -1 -1 -1 -1 -1]
  Discrete FIR Filter4 : DiscreteFir  FilterStructure=Direct form transposed  Coefficients=-1*[-1 1 -1 1 -1 -1 1 1 -1 -1 -1 -1 -1]
  Real-Imag to Complex2 : RealImagToComplex
  Out1 : Outport
  wires:
  Delay1/1 -> Discrete FIR Filter4/1
  Delay3/1 -> Real-Imag to Complex2/2
  Delay2/1 -> Real-Imag to Complex2/1
  Discrete FIR Filter4/1 -> Data Type Conversion1/1
  Delay4/1 -> Discrete FIR Filter3/1
  Discrete FIR Filter3/1 -> Data Type Conversion6/1
  Add3/1 -> Delay1/1
  Data Type Conversion6/1 -> Delay2/1
  Add2/1 -> Delay4/1
  Data Type Conversion1/1 -> Delay3/1
  Complex to Real-Imag2/1 -> Add3/1, Add2/1
  Complex to Real-Imag2/2 -> Add2/2, Add3/2
  Real-Imag to Complex2/1 -> Out1/1
  In1/1 -> Complex to Real-Imag2/1

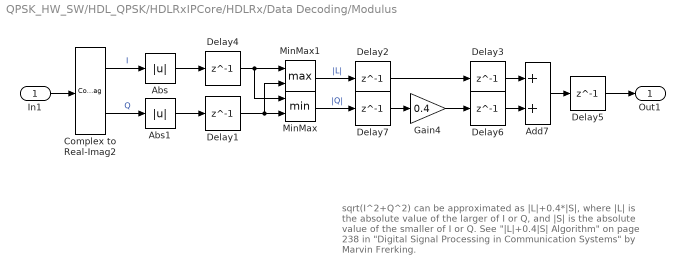
== system QPSK_HW_SW/HDL_QPSK/HDLRxIPCore/HDLRx/Data Decoding/Modulus ==
  note: sqrt(I^2+Q^2) can be approximated as |L|+0.4*|S|,
      | where |L| is the absolute value of the larger of I or Q,
      | and |S| is the absolute value of the smaller of I or Q.
      |
      | See "|L|+0.4|S| Algorithm" on page 238 in "Digital Signal
      | Processing in Communication Systems" by Marvin Frerking.
  In1 : Inport
  Abs : Abs
  Abs1 : Abs
  Add7 : Sum
  Complex to Real-Imag2 : ComplexToRealImag
  Delay{1..7} (7 alike) : Delay  DelayLength=1  InitialCondition=0
  Gain4 : Gain  Gain=0.4  OutDataTypeStr=fixdt(1,16,15)
  MinMax : MinMax  Inputs=2
  MinMax1 : MinMax  Function=max  Inputs=2
  Out1 : Outport
  wires:
  Complex to Real-Imag2/1 -> Abs/1  "I"
  Complex to Real-Imag2/2 -> Abs1/1  "Q"
  Delay3/1 -> Add7/1
  Delay5/1 -> Out1/1
  Delay6/1 -> Add7/2
  Delay4/1 -> MinMax/1, MinMax1/1
  Delay1/1 -> MinMax/2, MinMax1/2
  Delay2/1 -> Delay3/1
  Delay7/1 -> Gain4/1
  Add7/1 -> Delay5/1
  MinMax/1 -> Delay7/1  "|Q|"
  MinMax1/1 -> Delay2/1  "|L|"
  Gain4/1 -> Delay6/1
  Abs/1 -> Delay4/1
  Abs1/1 -> Delay1/1
  In1/1 -> Complex to Real-Imag2/1

== system QPSK_HW_SW/HDL_QPSK/HDLRxIPCore/HDLRx/Fine Frequency Compensation/Loop Filter ==
  note: Proportional-plus-Integrator Loop Filter,
      | Infinite DC Response to guarantee convergence
  e : Inport
  Data Type Conversion : DataTypeConversion  OutDataTypeStr=fixdt(1,16,15)
  Digital Filter : Subsystem
  K1 : Gain  Gain=K1  OutDataTypeStr=fixdt(1,16,15)
  K2 : Gain  Gain=K2  OutDataTypeStr=fixdt(1,32,32)
  Sum2 : Sum  OutDataTypeStr=fixdt(1,16,15)  SaturateOnIntegerOverflow=on
  Unit Delay2 : UnitDelay  SampleTime=-1
  v : Outport
  wires:
  Sum2/1 -> Unit Delay2/1
  Digital Filter/1(Out1) -> Data Type Conversion/1
  K1/1 -> Sum2/1
  Data Type Conversion/1 -> Sum2/2
  Unit Delay2/1 -> v/1
  e/1 -> K2/1, K1/1
  K2/1 -> Digital Filter/1(In1)

== system QPSK_HW_SW/HDL_QPSK/HDLRxIPCore/HDLRx/Fine Frequency Compensation/Phase Calculation ==
  Inc : Inport
  Add1 : Sum  OutDataTypeStr=fixdt(1,sdrzQPSKrxFPGA.WL_acc ,0)
  Constant : Constant  Value=sdrzQPSKrxFPGA.FFC_Const  OutDataTypeStr=fixdt(1,sdrzQPSKrxFPGA.WL_acc,0)  SampleTime=sdrzQPSKrxFPGA.Ts*sdrzQPSKrxFPGA.Upsampling/sdrzQPSKrxFPGA.Downsampling
  Integer Delay4 : Delay  DelayLength=1  InitialCondition=0  InputProcessing=Inherited
  Product : Product  OutDataTypeStr=fixdt(1,sdrzQPSKrxFPGA.WL_acc,0)
  Quart_Sin_Cos_LUT : Subsystem
  Real-Imag to Complex2 : RealImagToComplex
  Signal Specification : SignalSpecification  Dimensions=1
  phShift : Outport
  wires:
  Product/1 -> Add1/2
  Constant/1 -> Product/2
  Inc/1 -> Product/1
  Add1/1 -> Integer Delay4/1
  Integer Delay4/1 -> Add1/1, Signal Specification/1
  Quart_Sin_Cos_LUT/2(cosValue) -> Real-Imag to Complex2/1
  Quart_Sin_Cos_LUT/1(sineValue) -> Real-Imag to Complex2/2
  Real-Imag to Complex2/1 -> phShift/1
  Signal Specification/1 -> Quart_Sin_Cos_LUT/1(Phase)

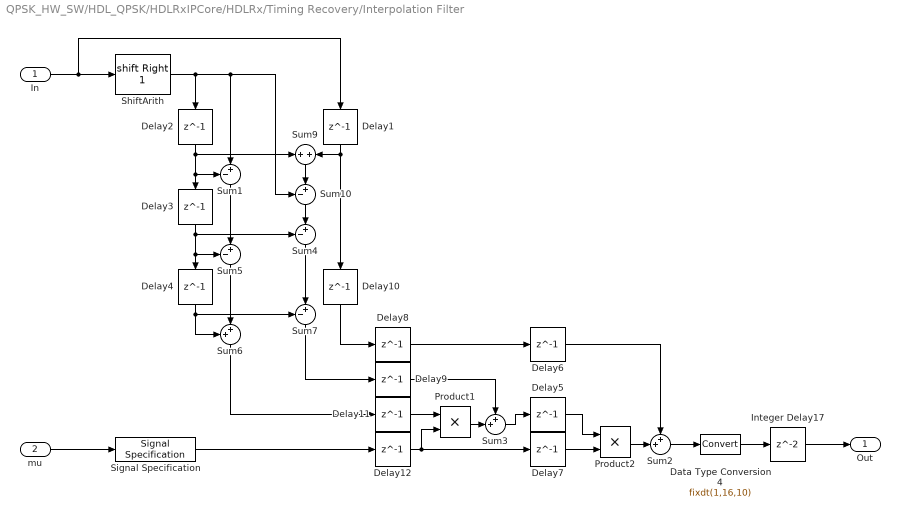
== system QPSK_HW_SW/HDL_QPSK/HDLRxIPCore/HDLRx/Timing Recovery/Interpolation Filter ==
  In : Inport
  mu : Inport  Port=2
  Data Type Conversion4 : DataTypeConversion  OutDataTypeStr=fixdt(1,16,10)
  Delay{1..12} (12 alike) : Delay  DelayLength=1  InitialCondition=0
  Integer Delay17 : Delay  InitialCondition=0  InputProcessing=Inherited
  Product1 : Product  OutDataTypeStr=fixdt(1,16,10)  RndMeth=Zero
  Product2 : Product  RndMeth=Zero
  ShiftArith : ArithShift  BitShiftNumber=1  BitShiftDirection=Right
  Signal Specification : SignalSpecification  Dimensions=1
  Sum{1,4..5,10} (4 alike) : Sum  Inputs=-+|
  Sum2 : Sum  Inputs=++|
  Sum3 : Sum  Inputs=++|  OutDataTypeStr=fixdt(1,16,10)
  Sum6 : Sum  Inputs=++|  OutDataTypeStr=fixdt(1,16,11)  SaturateOnIntegerOverflow=on
  Sum7 : Sum  Inputs=-+|  OutDataTypeStr=fixdt(1,16,10)
  Sum9 : Sum  Inputs=+|+
  Out : Outport
  wires:
  ShiftArith/1 -> Delay2/1, Sum1/2, Sum10/1
  Delay1/1 -> Sum9/2, Delay10/1
  Delay2/1 -> Sum9/1, Delay3/1, Sum1/1
  Sum10/1 -> Sum4/2
  Delay3/1 -> Delay4/1, Sum5/1, Sum4/1
  Sum1/1 -> Sum5/2
  Delay4/1 -> Sum6/1, Sum7/1
  Sum5/1 -> Sum6/2
  Sum4/1 -> Sum7/2
  Delay5/1 -> Product2/1
  Sum3/1 -> Delay5/1
  Product2/1 -> Sum2/2
  Product1/1 -> Sum3/2
  Sum2/1 -> Data Type Conversion4/1
  Delay11/1 -> Product1/1
  Delay9/1 -> Sum3/1
  Delay8/1 -> Delay6/1
  Delay12/1 -> Delay7/1, Product1/2
  Delay7/1 -> Product2/2
  Delay6/1 -> Sum2/1
  Delay10/1 -> Delay8/1
  Sum7/1 -> Delay9/1
  Sum6/1 -> Delay11/1
  mu/1 -> Signal Specification/1
  Integer Delay17/1 -> Out/1
  In/1 -> Delay1/1, ShiftArith/1
  Data Type Conversion4/1 -> Integer Delay17/1
  Sum9/1 -> Sum10/2
  Signal Specification/1 -> Delay12/1

== system QPSK_HW_SW/HDL_QPSK/HDLRxIPCore/HDLRx/Timing Recovery/Loop Filter ==
  note: Proportional-Plus-Integrator Loop Filter,
      | Infinite DC Response to guarantee convergence
  e : Inport
  Data Type Conversion17 : DataTypeConversion  OutDataTypeStr=fixdt(1,11,10)
  Delay1 : Delay  DelayLength=1  InitialCondition=0
  Delay2 : Delay  DelayLength=1  InitialCondition=0
  Delay4 : Delay  DelayLength=1  InitialCondition=0
  Digital Filter : Subsystem
  K1 : Gain  Gain=K1  OutDataTypeStr=fixdt(1,40,33)
  K2 : Gain  Gain=K2
  Sum2 : Sum  SaturateOnIntegerOverflow=on  InputSameDT=on
  v : Outport
  wires:
  e/1 -> Delay2/1
  Sum2/1 -> Data Type Conversion17/1
  Delay1/1 -> Sum2/1
  Delay4/1 -> Sum2/2
  Delay2/1 -> K1/1, K2/1
  Data Type Conversion17/1 -> v/1
  K2/1 -> Digital Filter/1(In1)
  Digital Filter/1(Out1) -> Delay4/1
  K1/1 -> Delay1/1

== system QPSK_HW_SW/HDL_QPSK/HDLTxIPCore/HDLTx/Data Generation & Packetization/Bit Pairing ==
  Serial In : Inport
  Bit Concat : hdlsllib/HDL Operations/Bit Concat  numInputs=2
      settings: SourceProductName=HDL Coder  SourceProductBaseCode=HD
  Delay1 : Delay  DelayLength=1
  Delay2 : Delay  DelayLength=1
  Downsample : DownSample  phase=1  RateOptions=Allow multirate processing
  Downsample1 : DownSample  RateOptions=Allow multirate processing
  Bit Pair : Outport
  wires:
  Downsample1/1 -> Delay1/1
  Serial In/1 -> Downsample1/1, Downsample/1
  Bit Concat/1 -> Bit Pair/1
  Downsample/1 -> Delay2/1
  Delay1/1 -> Bit Concat/2
  Delay2/1 -> Bit Concat/1

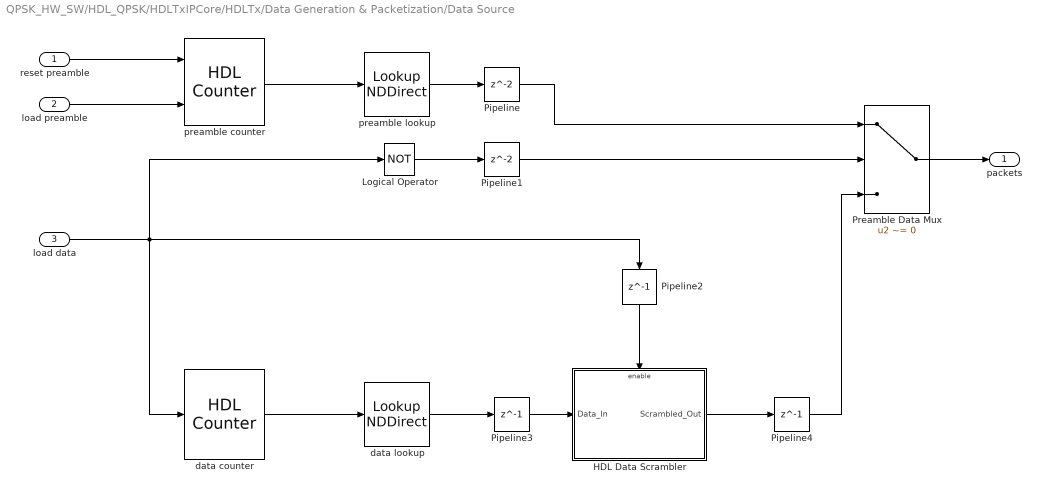
== system QPSK_HW_SW/HDL_QPSK/HDLTxIPCore/HDLTx/Data Generation & Packetization/Data Source ==
  reset preamble : Inport
  load preamble : Inport  Port=2
  load data : Inport  Port=3
  HDL Data Scrambler : Subsystem  TreatAsAtomicUnit=on
  Logical Operator : Logic  Operator=NOT  AllPortsSameDT=off  OutDataTypeStr=boolean
  Pipeline : Delay  InitialCondition=0
  Pipeline1 : Delay  InitialCondition=0
  Pipeline2 : Delay  DelayLength=1  InitialCondition=0
  Pipeline3 : Delay  DelayLength=1  InitialCondition=0
  Pipeline4 : Delay  DelayLength=1  InitialCondition=0
  Preamble Data Mux : Switch  Criteria=u2 ~= 0
  data counter : hdlsllib/HDL Operations/HDL Counter  CountType=Count limited  CountInit=0  CountStep=1  CountMax=17399  CountFromType=Initial value  CountFrom=0  CountResetPort=off  CountLoadPort=off  CountEnbPort=on  CountDirPort=off  CountDataType=Unsigned  CountWordLen=16  CountFracLen=0  CountSampTime=1
      settings: SourceProductName=HDL Coder  SourceProductBaseCode=HD
  data lookup : LookupNDDirect  NumberOfTableDimensions=1  Table=[qpsktxhdl.data]  DiagnosticForOutOfRangeInput=Error  TableDataTypeStr=boolean
  preamble counter : hdlsllib/HDL Operations/HDL Counter  CountType=Free running  CountInit=0  CountStep=1  CountMax=256  CountFromType=Initial value  CountFrom=0  CountResetPort=on  CountLoadPort=off  CountEnbPort=on  CountDirPort=off  CountDataType=Unsigned  CountWordLen=8  CountFracLen=0  CountSampTime=1
      settings: SourceProductName=HDL Coder  SourceProductBaseCode=HD
  preamble lookup : LookupNDDirect  NumberOfTableDimensions=1  Table=[qpsktxhdl.preamble]  DiagnosticForOutOfRangeInput=Error  TableDataTypeStr=boolean
  packets : Outport
  wires:
  load data/1 -> data counter/1, Pipeline2/1, Logical Operator/1
  Logical Operator/1 -> Pipeline1/1
  Pipeline2/1 -> HDL Data Scrambler/Enable
  Preamble Data Mux/1 -> packets/1
  Pipeline1/1 -> Preamble Data Mux/2
  Pipeline/1 -> Preamble Data Mux/1
  Pipeline4/1 -> Preamble Data Mux/3
  Pipeline3/1 -> HDL Data Scrambler/1(Data_In)
  preamble lookup/1 -> Pipeline/1
  HDL Data Scrambler/1(Scrambled_Out) -> Pipeline4/1
  data lookup/1 -> Pipeline3/1
  data counter/1 -> data lookup/1
  reset preamble/1 -> preamble counter/1
  load preamble/1 -> preamble counter/2
  preamble counter/1 -> preamble lookup/1

== system QPSK_HW_SW/HDL_QPSK/HDLRxIPCore/HDLRx/Coarse Frequency Compensation/luise_fixpt/Enabled Wire ==
  In1 : Inport
  Enable : EnablePort
  Data Type Conversion : DataTypeConversion  OutDataTypeStr=fixdt(1,sdrzQPSKrxFPGA.rad_WL,sdrzQPSKrxFPGA.rad_FL)
  Out1 : Outport  InitialOutput=0
  wires:
  In1/1 -> Data Type Conversion/1
  Data Type Conversion/1 -> Out1/1

== system QPSK_HW_SW/HDL_QPSK/HDLRxIPCore/HDLRx/Fine Frequency Compensation/Loop Filter/Digital Filter ==
  In1 : Inport
  Add1 : Sum  OutDataTypeStr=fixdt(1,32,32)
  Unit Delay1 : UnitDelay  SampleTime=-1
  Out1 : Outport
  wires:
  Unit Delay1/1 -> Add1/1
  Add1/1 -> Out1/1, Unit Delay1/1
  In1/1 -> Add1/2

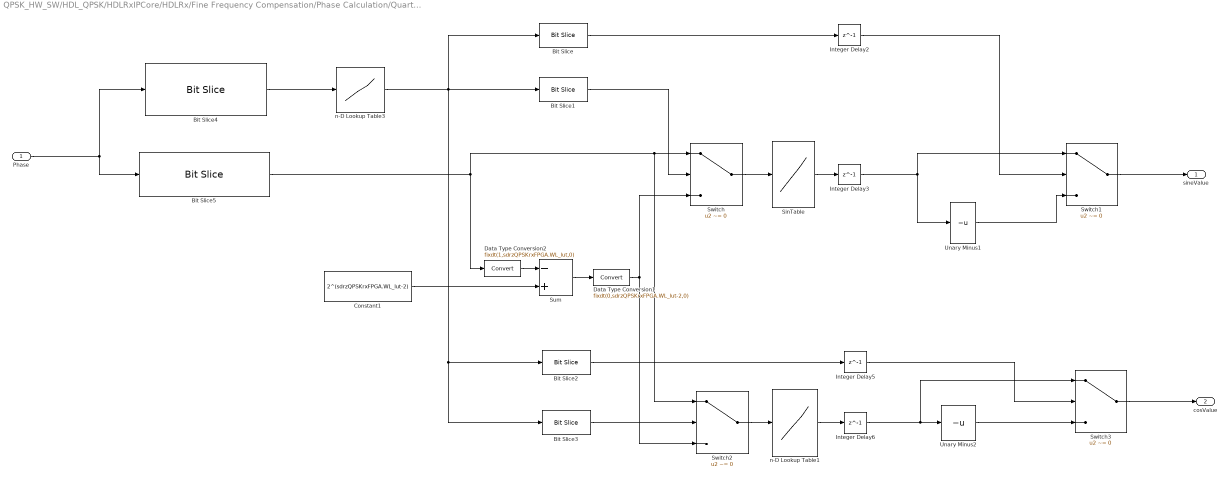
== system QPSK_HW_SW/HDL_QPSK/HDLRxIPCore/HDLRx/Fine Frequency Compensation/Phase Calculation/Quart_Sin_Cos_LUT ==
  Phase : Inport
  Bit Slice : hdlsllib/HDL Operations/Bit Slice  lidx=1  ridx=1
      settings: SourceProductName=HDL Coder  SourceProductBaseCode=HD
  Bit Slice1 : hdlsllib/HDL Operations/Bit Slice  lidx=0  ridx=0
      settings: SourceProductName=HDL Coder  SourceProductBaseCode=HD
  Bit Slice2 : hdlsllib/HDL Operations/Bit Slice  lidx=3  ridx=3
      settings: SourceProductName=HDL Coder  SourceProductBaseCode=HD
  Bit Slice3 : hdlsllib/HDL Operations/Bit Slice  lidx=2  ridx=2
      settings: SourceProductName=HDL Coder  SourceProductBaseCode=HD
  Bit Slice4 : hdlsllib/HDL Operations/Bit Slice  lidx=sdrzQPSKrxFPGA.WL_acc-1  ridx=sdrzQPSKrxFPGA.WL_acc-2
      settings: SourceProductName=HDL Coder  SourceProductBaseCode=HD
  Bit Slice5 : hdlsllib/HDL Operations/Bit Slice  lidx=sdrzQPSKrxFPGA.phMSB  ridx=sdrzQPSKrxFPGA.phLSB
      settings: SourceProductName=HDL Coder  SourceProductBaseCode=HD
  Constant1 : Constant  Value=2^(sdrzQPSKrxFPGA.WL_lut-2)  OutDataTypeStr=fixdt(1,sdrzQPSKrxFPGA.WL_lut,0)  SampleTime=-1
  Data Type Conversion1 : DataTypeConversion  OutDataTypeStr=fixdt(0,sdrzQPSKrxFPGA.WL_lut-2,0)
  Data Type Conversion2 : DataTypeConversion  OutDataTypeStr=fixdt(1,sdrzQPSKrxFPGA.WL_lut,0)
  Integer Delay{2..3,5..6} (4 alike) : Delay  DelayLength=1  InitialCondition=0  InputProcessing=Inherited
  SinTable : Lookup_n-D  NumberOfTableDimensions=1  LookupTableObject=''  BreakpointsForDimension1=[0:length(sdrzQPSKrxFPGA.sin_tbl)-1]  BreakpointsForDimension2=[1:2]  BreakpointsForDimension3=[5, 7]  BreakpointsForDimension1FirstPoint=10  BreakpointsForDimension2FirstPoint=10  BreakpointsForDimension1Spacing=12  BreakpointsForDimension2Spacing=12  IndexSearchMethod=Evenly spaced points  Table=sdrzQPSKrxFPGA.sin_tbl  InterpMethod=Flat  DiagnosticForOutOfRangeInput=Error  InternalRulePriority=Speed  OutDataTypeStr=fixdt(1, sdrzQPSKrxFPGA.WL_out,sdrzQPSKrxFPGA.WL_out-2)  SaturateOnIntegerOverflow=on  InputSameDT=on
  Sum : Sum  Inputs=-+  OutDataTypeStr=fixdt(1,sdrzQPSKrxFPGA.WL_lut,0)  InputSameDT=on
  Switch{,1..3} (4 alike) : Switch  Criteria=u2 ~= 0  SaturateOnIntegerOverflow=on  InputSameDT=on
  Unary Minus1 : UnaryMinus
  Unary Minus2 : UnaryMinus
  n-D Lookup Table1 : Lookup_n-D  NumberOfTableDimensions=1  LookupTableObject=''  BreakpointsForDimension1=[0:length(sdrzQPSKrxFPGA.cos_tbl)-1]  BreakpointsForDimension2=[1:2]  BreakpointsForDimension3=[5, 7]  BreakpointsForDimension1FirstPoint=10  BreakpointsForDimension2FirstPoint=10  BreakpointsForDimension1Spacing=12  BreakpointsForDimension2Spacing=12  IndexSearchMethod=Evenly spaced points  Table=sdrzQPSKrxFPGA.cos_tbl  InterpMethod=Flat  DiagnosticForOutOfRangeInput=Error  InternalRulePriority=Speed  OutDataTypeStr=fixdt(1,sdrzQPSKrxFPGA.WL_out,sdrzQPSKrxFPGA.WL_out-2)  SaturateOnIntegerOverflow=on  InputSameDT=on
  n-D Lookup Table3 : Lookup_n-D  NumberOfTableDimensions=1  LookupTableObject=''  BreakpointsForDimension1=[0:3]  BreakpointsForDimension2=[1:2]  BreakpointsForDimension3=[5, 7]  BreakpointsForDimension1FirstPoint=10  BreakpointsForDimension2FirstPoint=10  BreakpointsForDimension1Spacing=12  BreakpointsForDimension2Spacing=12  IndexSearchMethod=Evenly spaced points  Table=[15 2 5 8]  InterpMethod=Flat  DiagnosticForOutOfRangeInput=Error  InternalRulePriority=Speed  OutDataTypeStr=fixdt(0,4,0)  SaturateOnIntegerOverflow=on  InputSameDT=on
  sineValue : Outport
  cosValue : Outport  Port=2
  wires:
  Phase/1 -> Bit Slice5/1, Bit Slice4/1
  Constant1/1 -> Sum/2
  SinTable/1 -> Integer Delay3/1
  Switch2/1 -> n-D Lookup Table1/1
  Bit Slice4/1 -> n-D Lookup Table3/1
  Integer Delay5/1 -> Switch3/2
  Unary Minus1/1 -> Switch1/3
  Bit Slice3/1 -> Switch2/2
  Data Type Conversion2/1 -> Sum/1
  n-D Lookup Table1/1 -> Integer Delay6/1
  Sum/1 -> Data Type Conversion1/1
  Integer Delay3/1 -> Switch1/1, Unary Minus1/1
  Bit Slice5/1 -> Data Type Conversion2/1, Switch/1, Switch2/1
  Data Type Conversion1/1 -> Switch2/3, Switch/3
  Bit Slice/1 -> Integer Delay2/1
  Switch1/1 -> sineValue/1
  Bit Slice1/1 -> Switch/2
  Integer Delay6/1 -> Switch3/1, Unary Minus2/1
  Switch3/1 -> cosValue/1
  Unary Minus2/1 -> Switch3/3
  Bit Slice2/1 -> Integer Delay5/1
  Switch/1 -> SinTable/1
  Integer Delay2/1 -> Switch1/2
  n-D Lookup Table3/1 -> Bit Slice1/1, Bit Slice/1, Bit Slice2/1, Bit Slice3/1
